simulink model "fxpdemo_probe"  (Simulink 5.0)
settings: Solver=ode45  StartTime=0.0  StopTime=10.0  RelTol=1e-3
settings Model: Creator=jretik  LastModifiedBy=jretik  ExtModeAutoUpdateStatusClock=off  SignalLoggingName=logsOut  ConditionalExecOptimization=on  ZeroCrossControl=UseLocalSettings  RTWMathFcnLibMatFile=iso_c_tmw.mat  RTWOptions="-aEnforceIntegerDowncast=1 -aFoldNonRolledExpr=1 -aInlineInvariantSignals=1 -aInlineParameters=0 -aLocalBlockOutputs=1 -aRollThreshold=5 -aRTWVerbose=1 -aGenerateReport=0 -aForceParamTrailComments=0 -aGenerateComments=1 -aIgnoreCustomStorageClasses=1 -aIncHierarchyInIds=0 -aMaxRTWIdLen=31 -aShowEliminatedStatements=0 -aReadOnly=0 -aTargetFcnLib=\"iso_c_tmw.mat\" -aIncDataTypeInIds=0 -aPrefixModelToSubsysFcnNames=1 -aInlinedPrmAccess=\"Literals\" -aGenerateFullHeader=1 -aIsPILTarget=0 -aLogVarNameModifier=\"rt_\" -aExtMode=0 -aExtModeStaticAlloc=0 -aExtModeTesting=0 -aExtModeStaticAllocSize=1000000 -aExtModeTransport=0  -aInlineParameters=0 -aExtModeTransport=\"tcpip\" -aInlineParameters=0 -aInlineParameters=0 -aInlineParameters=0 -aInlineParameters=0"

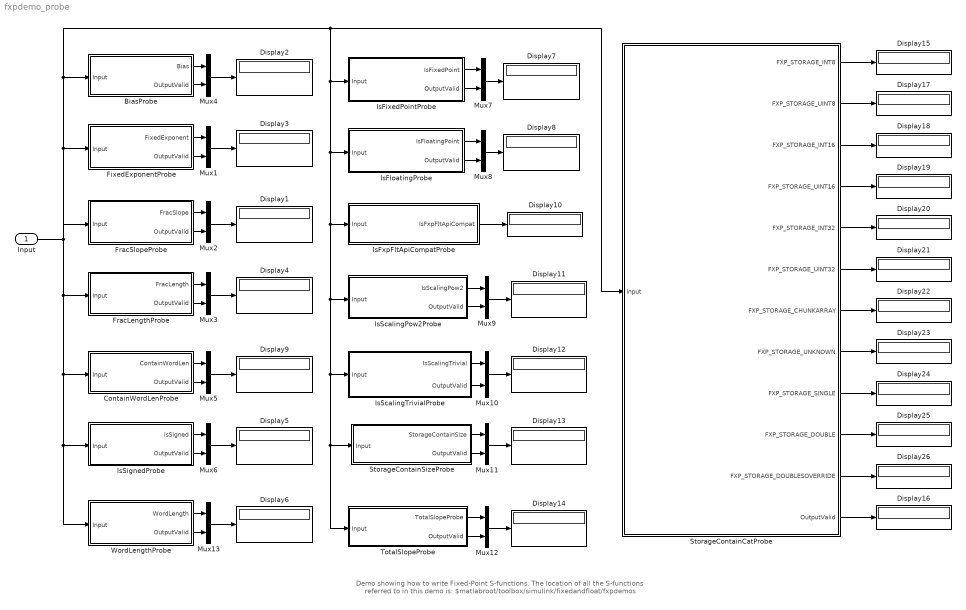
== system fxpdemo_probe ==
  note: Demo showing how to write Fixed-Point S-functions.  The location of all the S-functions referred
      | to in this demo is: $matlabroot/toolbox/simulink/fixedandfloat/fxpdemos
  Input : Inport  ShowAdditionalParam=on  DataType=Specify via dialog  OutDataType=sfix(33)  OutScaling=[1.1*2^-3 10]
  BiasProbe : Subsystem
  ContainWordLenProbe : Subsystem
  Display{1..26} (26 alike) : Display
  FixedExponentProbe : Subsystem
  FracLengthProbe : Subsystem
  FracSlopeProbe : Subsystem
  IsFixedPointProbe : Subsystem
  IsFloatingProbe : Subsystem
  IsFxpFltApiCompatProbe : Subsystem
  IsScalingPow2Probe : Subsystem
  IsScalingTrivialProbe : Subsystem
  IsSignedProbe : Subsystem
  Mux{1..13} (13 alike) : Mux  Inputs=2
  StorageContainCatProbe : Subsystem
  StorageContainSizeProbe : Subsystem
  "TotalSlopeProbe " : Subsystem
  WordLengthProbe : Subsystem
  wires:
  Mux5/1 -> Display9/1
  Mux3/1 -> Display4/1
  Mux2/1 -> Display1/1
  Mux1/1 -> Display3/1
  Mux4/1 -> Display2/1
  Input/1 -> FixedExponentProbe/1(Input), BiasProbe/1(Input), IsFixedPointProbe/1(Input), IsFloatingProbe/1(Input), IsFxpFltApiCompatProbe/1(Input), IsScalingPow2Probe/1(Input), IsScalingTrivialProbe/1(Input), StorageContainSizeProbe/1(Input), "TotalSlopeProbe "/1(Input), StorageContainCatProbe/1(Input), FracSlopeProbe/1(Input), FracLengthProbe/1(Input), ContainWordLenProbe/1(Input), IsSignedProbe/1(Input), WordLengthProbe/1(Input)
  Mux6/1 -> Display5/1
  IsSignedProbe/1(IsSigned) -> Mux6/1
  IsSignedProbe/2(OutputValid) -> Mux6/2
  Mux13/1 -> Display6/1
  WordLengthProbe/1(WordLength) -> Mux13/1
  WordLengthProbe/2(OutputValid) -> Mux13/2
  Mux7/1 -> Display7/1
  IsFixedPointProbe/1(IsFixedPoint) -> Mux7/1
  IsFixedPointProbe/2(OutputValid) -> Mux7/2
  IsFloatingProbe/1(IsFloatingPoint) -> Mux8/1
  IsFloatingProbe/2(OutputValid) -> Mux8/2
  IsFxpFltApiCompatProbe/1(IsFxpFltApiCompat) -> Display10/1
  Mux9/1 -> Display11/1
  IsScalingPow2Probe/1(IsScalingPow2) -> Mux9/1
  IsScalingPow2Probe/2(OutputValid) -> Mux9/2
  Mux10/1 -> Display12/1
  IsScalingTrivialProbe/1(IsScalingTrivial) -> Mux10/1
  Mux11/1 -> Display13/1
  StorageContainSizeProbe/1(StorageContainSize) -> Mux11/1
  StorageContainSizeProbe/2(OutputValid) -> Mux11/2
  Mux12/1 -> Display14/1
  "TotalSlopeProbe "/1(TotalSlopeProbe) -> Mux12/1
  "TotalSlopeProbe "/2(OutputValid) -> Mux12/2
  BiasProbe/1(Bias) -> Mux4/1
  BiasProbe/2(OutputValid) -> Mux4/2
  FixedExponentProbe/1(FixedExponent) -> Mux1/1
  FixedExponentProbe/2(OutputValid) -> Mux1/2
  FracSlopeProbe/1(FracSlope) -> Mux2/1
  FracSlopeProbe/2(OutputValid) -> Mux2/2
  FracLengthProbe/1(FracLength) -> Mux3/1
  FracLengthProbe/2(OutputValid) -> Mux3/2
  ContainWordLenProbe/1(ContainWordLen) -> Mux5/1
  ContainWordLenProbe/2(OutputValid) -> Mux5/2
  StorageContainCatProbe/1(FXP_STORAGE_INT8) -> Display15/1
  StorageContainCatProbe/2(FXP_STORAGE_UINT8) -> Display17/1
  StorageContainCatProbe/3(FXP_STORAGE_INT16) -> Display18/1
  StorageContainCatProbe/4(FXP_STORAGE_UINT16) -> Display19/1
  StorageContainCatProbe/5(FXP_STORAGE_INT32) -> Display20/1
  StorageContainCatProbe/6(FXP_STORAGE_UINT32) -> Display21/1
  StorageContainCatProbe/7(FXP_STORAGE_CHUNKARRAY) -> Display22/1
  StorageContainCatProbe/8(FXP_STORAGE_UNKNOWN) -> Display23/1
  StorageContainCatProbe/9(FXP_STORAGE_SINGLE) -> Display24/1
  StorageContainCatProbe/10(FXP_STORAGE_DOUBLE) -> Display25/1
  StorageContainCatProbe/11(FXP_STORAGE_DOUBLESOVERRIDE) -> Display26/1
  StorageContainCatProbe/12(OutputValid) -> Display16/1
  Mux8/1 -> Display8/1
  IsScalingTrivialProbe/2(OutputValid) -> Mux10/2

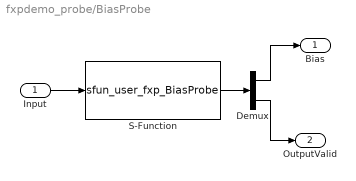
== system fxpdemo_probe/BiasProbe ==
  Input : Inport
  Demux : Demux  Outputs=2
  S-Function : S-Function  FunctionName=sfun_user_fxp_BiasProbe
  Bias : Outport
  OutputValid : Outport  Port=2
  wires:
  Input/1 -> S-Function/1
  S-Function/1 -> Demux/1
  Demux/1 -> Bias/1
  Demux/2 -> OutputValid/1

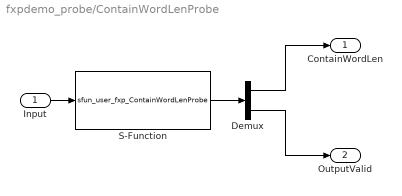
== system fxpdemo_probe/ContainWordLenProbe ==
  Input : Inport
  Demux : Demux  Outputs=2
  S-Function : S-Function  FunctionName=sfun_user_fxp_ContainWordLenProbe
  ContainWordLen : Outport
  OutputValid : Outport  Port=2
  wires:
  Demux/1 -> ContainWordLen/1
  Demux/2 -> OutputValid/1
  S-Function/1 -> Demux/1
  Input/1 -> S-Function/1

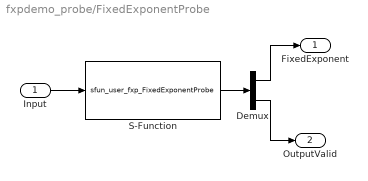
== system fxpdemo_probe/FixedExponentProbe ==
  Input : Inport
  Demux : Demux  Outputs=2
  S-Function : S-Function  FunctionName=sfun_user_fxp_FixedExponentProbe
  FixedExponent : Outport
  OutputValid : Outport  Port=2
  wires:
  Demux/2 -> OutputValid/1
  Demux/1 -> FixedExponent/1
  S-Function/1 -> Demux/1
  Input/1 -> S-Function/1

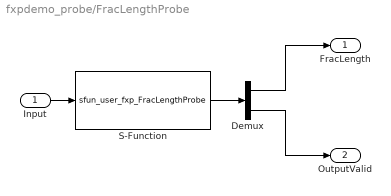
== system fxpdemo_probe/FracLengthProbe ==
  Input : Inport
  Demux : Demux  Outputs=2
  S-Function : S-Function  FunctionName=sfun_user_fxp_FracLengthProbe
  FracLength : Outport
  OutputValid : Outport  Port=2
  wires:
  Input/1 -> S-Function/1
  S-Function/1 -> Demux/1
  Demux/2 -> OutputValid/1
  Demux/1 -> FracLength/1

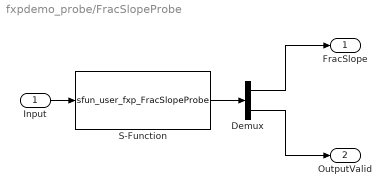
== system fxpdemo_probe/FracSlopeProbe ==
  Input : Inport
  Demux : Demux  Outputs=2
  S-Function : S-Function  FunctionName=sfun_user_fxp_FracSlopeProbe
  FracSlope : Outport
  OutputValid : Outport  Port=2
  wires:
  Demux/1 -> FracSlope/1
  Demux/2 -> OutputValid/1
  S-Function/1 -> Demux/1
  Input/1 -> S-Function/1

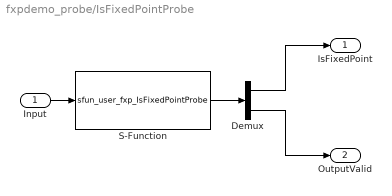
== system fxpdemo_probe/IsFixedPointProbe ==
  Input : Inport
  Demux : Demux  Outputs=2
  S-Function : S-Function  FunctionName=sfun_user_fxp_IsFixedPointProbe
  IsFixedPoint : Outport
  OutputValid : Outport  Port=2
  wires:
  Input/1 -> S-Function/1
  S-Function/1 -> Demux/1
  Demux/2 -> OutputValid/1
  Demux/1 -> IsFixedPoint/1

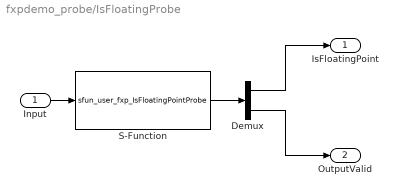
== system fxpdemo_probe/IsFloatingProbe ==
  Input : Inport
  Demux : Demux  Outputs=2
  S-Function : S-Function  FunctionName=sfun_user_fxp_IsFloatingPointProbe
  IsFloatingPoint : Outport
  OutputValid : Outport  Port=2
  wires:
  Demux/1 -> IsFloatingPoint/1
  Demux/2 -> OutputValid/1
  S-Function/1 -> Demux/1
  Input/1 -> S-Function/1

== system fxpdemo_probe/IsFxpFltApiCompatProbe ==
  Input : Inport
  S-Function : S-Function  FunctionName=sfun_user_fxp_IsFxpFltApiCompatProbe
  IsFxpFltApiCompat : Outport
  wires:
  Input/1 -> S-Function/1
  S-Function/1 -> IsFxpFltApiCompat/1

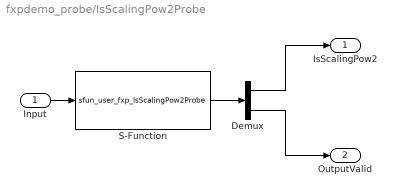
== system fxpdemo_probe/IsScalingPow2Probe ==
  Input : Inport
  Demux : Demux  Outputs=2
  S-Function : S-Function  FunctionName=sfun_user_fxp_IsScalingPow2Probe
  IsScalingPow2 : Outport
  OutputValid : Outport  Port=2
  wires:
  Input/1 -> S-Function/1
  S-Function/1 -> Demux/1
  Demux/2 -> OutputValid/1
  Demux/1 -> IsScalingPow2/1

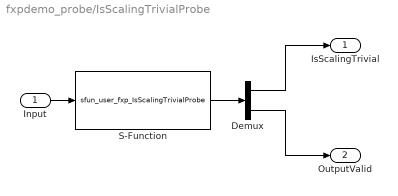
== system fxpdemo_probe/IsScalingTrivialProbe ==
  Input : Inport
  Demux : Demux  Outputs=2
  S-Function : S-Function  FunctionName=sfun_user_fxp_IsScalingTrivialProbe
  IsScalingTrivial : Outport
  OutputValid : Outport  Port=2
  wires:
  Demux/1 -> IsScalingTrivial/1
  Demux/2 -> OutputValid/1
  S-Function/1 -> Demux/1
  Input/1 -> S-Function/1

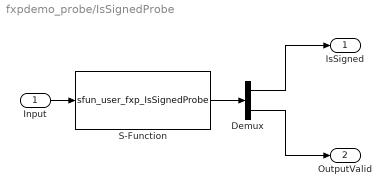
== system fxpdemo_probe/IsSignedProbe ==
  Input : Inport
  Demux : Demux  Outputs=2
  S-Function : S-Function  FunctionName=sfun_user_fxp_IsSignedProbe
  IsSigned : Outport
  OutputValid : Outport  Port=2
  wires:
  Input/1 -> S-Function/1
  S-Function/1 -> Demux/1
  Demux/2 -> OutputValid/1
  Demux/1 -> IsSigned/1

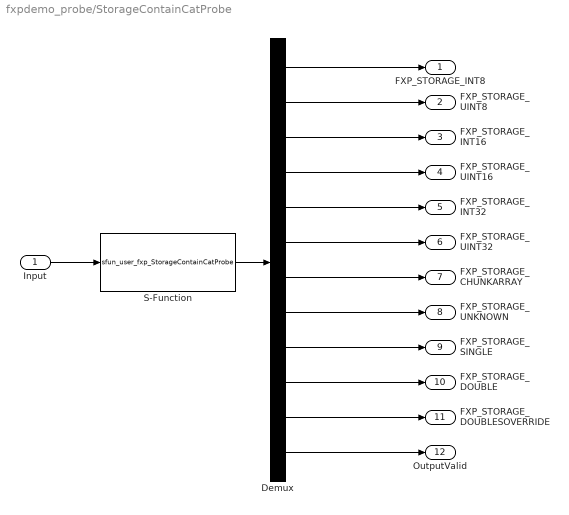
== system fxpdemo_probe/StorageContainCatProbe ==
  Input : Inport
  Demux : Demux  Outputs=12
  S-Function : S-Function  FunctionName=sfun_user_fxp_StorageContainCatProbe
  FXP_STORAGE_INT8 : Outport
  FXP_STORAGE_UINT8 : Outport  Port=2
  FXP_STORAGE_INT16 : Outport  Port=3
  FXP_STORAGE_UINT16 : Outport  Port=4
  FXP_STORAGE_INT32 : Outport  Port=5
  FXP_STORAGE_UINT32 : Outport  Port=6
  FXP_STORAGE_CHUNKARRAY : Outport  Port=7
  FXP_STORAGE_UNKNOWN : Outport  Port=8
  FXP_STORAGE_SINGLE : Outport  Port=9
  FXP_STORAGE_DOUBLE : Outport  Port=10
  FXP_STORAGE_DOUBLESOVERRIDE : Outport  Port=11
  OutputValid : Outport  Port=12
  wires:
  Input/1 -> S-Function/1
  S-Function/1 -> Demux/1
  Demux/2 -> FXP_STORAGE_UINT8/1
  Demux/1 -> FXP_STORAGE_INT8/1
  Demux/3 -> FXP_STORAGE_INT16/1
  Demux/4 -> FXP_STORAGE_UINT16/1
  Demux/5 -> FXP_STORAGE_INT32/1
  Demux/6 -> FXP_STORAGE_UINT32/1
  Demux/11 -> FXP_STORAGE_DOUBLESOVERRIDE/1
  Demux/10 -> FXP_STORAGE_DOUBLE/1
  Demux/9 -> FXP_STORAGE_SINGLE/1
  Demux/8 -> FXP_STORAGE_UNKNOWN/1
  Demux/7 -> FXP_STORAGE_CHUNKARRAY/1
  Demux/12 -> OutputValid/1

== system fxpdemo_probe/StorageContainSizeProbe ==
  Input : Inport
  Demux : Demux  Outputs=2
  S-Function : S-Function  FunctionName=sfun_user_fxp_StorageContainSizeProbe
  StorageContainSize : Outport
  OutputValid : Outport  Port=2
  wires:
  Input/1 -> S-Function/1
  S-Function/1 -> Demux/1
  Demux/2 -> OutputValid/1
  Demux/1 -> StorageContainSize/1

== system fxpdemo_probe/TotalSlopeProbe  ==
  Input : Inport
  Demux : Demux  Outputs=2
  S-Function : S-Function  FunctionName=sfun_user_fxp_TotalSlopeProbe
  TotalSlopeProbe : Outport
  OutputValid : Outport  Port=2
  wires:
  Demux/1 -> TotalSlopeProbe/1
  Demux/2 -> OutputValid/1
  S-Function/1 -> Demux/1
  Input/1 -> S-Function/1

== system fxpdemo_probe/WordLengthProbe ==
  Input : Inport
  Demux : Demux  Outputs=2
  S-Function : S-Function  FunctionName=sfun_user_fxp_WordLengthProbe
  WordLength : Outport
  OutputValid : Outport  Port=2
  wires:
  Demux/1 -> WordLength/1
  Demux/2 -> OutputValid/1
  S-Function/1 -> Demux/1
  Input/1 -> S-Function/1
